simulink model "test6_namechange_orig"  (R2018a)
settings: Solver=VariableStepAuto  StartTime=0.0  StopTime=10.0  RelTol=1e-3
settings Model: Creator=monika  LastModifiedBy=monika

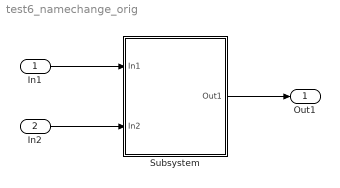
== system test6_namechange_orig ==
  In1 : Inport
  In2 : Inport  Port=2
  Subsystem : Subsystem
  Out1 : Outport
  wires:
  Subsystem/1(Out1) -> Out1/1
  In1/1 -> Subsystem/1(In1)
  In2/1 -> Subsystem/2(In2)

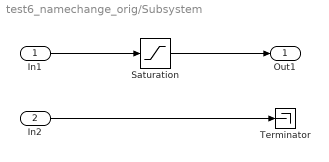
== system test6_namechange_orig/Subsystem ==
  In1 : Inport
  In2 : Inport  Port=2
  Saturation : Saturate
  Terminator : Terminator
  Out1 : Outport
  wires:
  In2/1 -> Terminator/1
  In1/1 -> Saturation/1
  Saturation/1 -> Out1/1
